simulink model "original_sim_bandpass_singleBand"  (R2024b)
settings: Solver=FixedStepDiscrete  StartTime=0.0  StopTime=(size(sm_EEG_data,1)-1)/sm.p.EEG.sr  RelTol=1e-3  EnableMultiTasking=on
values from neighbouring files (symbols this model uses):
  sm =     [reference_output.mat]
undefined symbols (not defined in the file or in its folder): fdesignblkfcn, gcbh
libraries: dspsrcs4 x1
settings Model: Creator=ronens  LastModifiedBy=hardeep
settings SolverCC: AlgebraicLoopSolver=TrustRegion
settings DataIOCC: LimitDataPoints=on  SaveFormat=Array  SignalLoggingSaveFormat=ModelDataLogs  ReturnWorkspaceOutputs=off
settings OptimizationCC: ExpressionDepthLimit=2147483647  LifeSpan=inf
settings DebuggingCC: UnderspecifiedInitializationDetection=Classic  MergeDetectMultiDrivingBlocksExec=none  SolverPrmCheckMsg=warning  ParameterPrecisionLossMsg=none  FcnCallInpInsideContextMsg=warning  UnconnectedInputMsg=warning  UnconnectedOutputMsg=warning  UnconnectedLineMsg=warning  StateNameClashWarn=warning  SFUnexpectedBacktrackingDiag=warning  SFNoUnconditionalDefaultTransitionDiag=warning  SFExecutionAtInitializationDiag=none  ArithmeticOperatorsInVariantConditions=warning
settings HardwareCC: ProdBitPerPointer=32  ProdBitPerSizeT=32  ProdBitPerPtrDiffT=32  ProdLargestAtomicFloat=None  ProdIntDivRoundTo=Undefined  ProdEndianess=Unspecified  ProdWordSize=32  ProdHWDeviceType=32-bit Generic
settings ModelReferenceCC: EnableRefExpFcnMdlSchedulingChecks=on  PropagateSignalLabelsOutOfModel=off
settings SFSimCC: SimUseLocalCustomCode=off  CustomCodeUndefinedFunction=UseInterfaceOnly
settings RTWCC: RTWUseLocalCustomCode=off  GPUComputeCapability=3.5
settings CodeAppCC: StateflowObjectComments=on
settings GRTTargetCC: TargetLangStandard=C89/C90 (ANSI)
settings ConfigComp: CovMetricSettings=dw  CovSaveCumulativeToWorkspaceVar=on  CovSaveSingleToWorkspaceVar=on  CovExternalEMLEnable=off
settings SimscapeCC: SimscapeNormalizeSystem=off
settings ConfigurationSet: Description=SimMechanics 2G

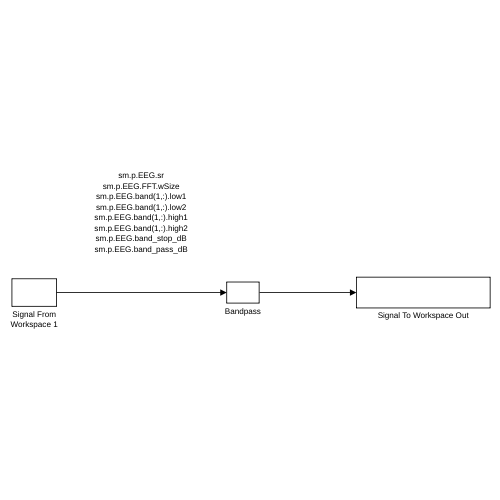
[thumbnail: Simulink's stored preview of the top-level diagram]
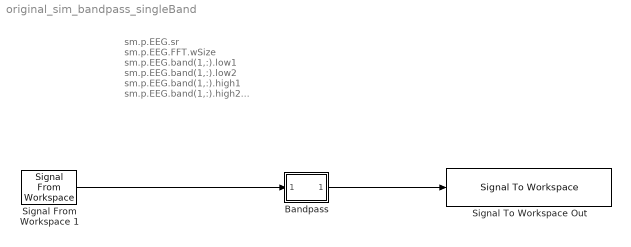
== system original_sim_bandpass_singleBand ==
  note: sm.p.EEG.sr
      | sm.p.EEG.FFT.wSize
      | sm.p.EEG.band(1,:).low1
      | sm.p.EEG.band(1,:).low2
      | sm.p.EEG.band(1,:).high1
      | sm.p.EEG.band(1,:).high2
      | sm.p.EEG.band_stop_dB
      | sm.p.EEG.band_pass_dB
  Bandpass : Subsystem
  Signal From Workspace 1 : dspsrcs4/Signal From Workspace  X=sm_EEG_data  Ts=1/sm.p.EEG.sr  nsamps=1  OutputAfterFinalValue=Setting to zero  ignoreOrWarnInputAndFrameLengths=off  OutputFrames=on
  Signal To Workspace Out : SignalToWorkspace  VariableName=Bandpass_singleBand
      settings: CopyFcn=dspblkcopystw(gcbh);
  wires:
  Signal From Workspace 1/1 -> Bandpass/1(In1)
  Bandpass/1(Out1) -> Signal To Workspace Out/1

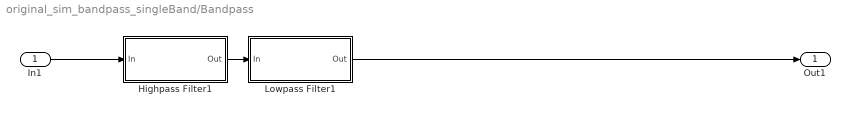
== system original_sim_bandpass_singleBand/Bandpass ==
  In1 : Inport
  Highpass Filter1 : Subsystem  DialogController=fdesignblkfcn  InitFcn=fdesignblkfcn(gcbh, {'InitFcn'});  mask(Highpass Filter){}
      mask help: Design a highpass filter
      settings: CopyFcn=fdesignblkfcn(gcbh, {'CopyFcn'});
      mask Help: helpview(mapfilelocation('dsp'), 'dsphighpassfilter');
      mask Display: disp('Highpass')
  Lowpass Filter1 : Subsystem  DialogController=fdesignblkfcn  InitFcn=fdesignblkfcn(gcbh, {'InitFcn'});  mask(Lowpass Filter){}
      mask help: Design a lowpass filter
      settings: CopyFcn=fdesignblkfcn(gcbh, {'CopyFcn'});
      mask Help: helpview(mapfilelocation('dsp'), 'dsplowpassfilter');
      mask Display: disp('Lowpass')
  Out1 : Outport
  wires:
  In1/1 -> Highpass Filter1/1(In)
  Highpass Filter1/1(Out) -> Lowpass Filter1/1(In)
  Lowpass Filter1/1(Out) -> Out1/1

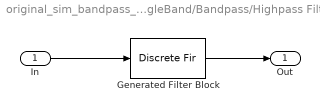
== system original_sim_bandpass_singleBand/Bandpass/Highpass Filter1 ==
  In : Inport
  Generated Filter Block : DiscreteFir  Tag=BlockMethodSubSystem  Coefficients=[-0.00840141778639717091 0.0173152224167967689 0.00308884947939271895 -0.00256762501130670907 -0.00423142192173075072 -0.00412026657980465571 -0.00329310593463389128 -0.002262732561662414 -0.00125968485465549444 -0.000392684840722325548 0.000304955573172563323 0.000822116755893660938 0.00117292528572729925 0.00137046595797921263 0.00144020225152880648 0.00139972588165432278 0.00127632771193091879 0.00108595288663199075 0.000854103588177903888 0.000594267545754096531 0.000327694684087062886 6.38551808909070077e-05 -0.000179450724560961872 -0.000397874081475507052 -0.000577963879948238429 -0.000719776889684668048 -0.000814672778546917699 -0.000866690567111298824 -0.000870392468345223169 -0.000834408096741966242 -0.000756342536848797205 -0.000647695094384184711 -0.000508513373527671726 -0.000352052829416214417 -0.000179389813557604598 -6.03349057744724519e-06 0.000167995555248989494 0.000327549877530480251 0.000473373899657685937 0.000591363324463213482 0.000685218342133664306 0.000741329035878340653 0.000768585479969400827 0.000753109204614785797 0.000709989097617417142 0.000626074902749358566 0.000518403169583120838 0.000387532180141191625 0.000223486800967541188 8.11274228046873498e-05 -0.000115389367192012801 -0.00025834783697307155 -0.000417485752251392625 -0.000565245925697868646 -0.000663489424197992125 -0.000742195313648855441 -0.000802778125940541609 -0.000807484686633235427 -0.000770219657810799476 -0.000711631558497011012 -0.000619998931755313823 -0.000483050872794562052 -0.000321413988640333764 -0.000153717015526360409 2.27220941756313879e-05 0.000210824767849350427 0.00039636524325277955 0.00055828007153160364 0.000690912002654363614 0.000797140998280385224 0.000875342473615355683 0.000912254358274695756 0.000900890166260798642 0.0008416310845922925 0.000745167556431057293 0.000616216536435795249 0.000457526778234206011 0.000268148897373869123 5.91646691704717247e-05 -0.000157866268265354696 -0.000366404857881273585 -0.000559796517825759368 -0.000730065774504567153 -0.00087460992705030321 -0.000981106285025435797 -0.00104421636832933225 -0.00105372525111916641 -0.00101210867575669741 -0.000919233909846757058 -0.000785414510046180542 -0.000610381701853770532 -0.000406780191843504548 -0.000173303851576987235 7.20373868736900541e-05 0.00032448590556910246 0.000564583909527311334 0.000778948373045466164 0.000965020151494673387 0.00109860528816741799 0.00119531980427785246 0.00122974161480201953 0.00120996458749239762 0.00113578507003964688 0.000997595080588046645 0.00080991362702319302 0.000580730320013465276 0.000313104306345794953 2.7668199553746984e-05 -0.000260607543396719867 -0.00054613423249910871 -0.000812759539448379875 -0.00104353866549433054 -0.00123218715350877236 -0.00137044349611684102 -0.00144309434064109434 -0.00144615789305872289 -0.00138121076942770179 -0.0012489288980708326 -0.001050081849674757 -0.000796785231903415791 -0.000502178253391383873 -0.000178960051172325933 0.000163224766678344001 0.000505737826522577186 0.000830861151816729448 0.00112283471959526409 0.00137186034084307829 0.00156132287412795532 0.00167952107584457954 0.00171702472149959785 0.00167415493664422785 0.00154974850149049224 0.001348980083380775 0.00107592528674645875 0.000746673324626800808 0.000374655135267273995 -2.16159478310621574e-05 -0.00042863836990482667 -0.000824381222395672306 -0.00119351166901265969 -0.00151019214123175919 -0.00176512000639446917 -0.00193998548851638465 -0.00202938824178094555 -0.00202275738797201652 -0.001915866871585006 -0.0017167889668052343 -0.00142672770768961441 -0.0010660049780923872 -0.000644129787264740715 -0.000178970697292878822 0.000303711730957656944 0.000786656921706672301 0.00124129009773345689 0.001646399374701221 0.00198576971536819531 0.00223936228102286162 0.00239129921621168522 0.00243491905326593009 0.0023616376574131224 0.0021716729037668729 0.0018740983339220643 0.00148042770867760128 0.00100322029275638921 0.0004662268872081259 -0.000107610602182091865 -0.000692898192660682281 ...(+8639 chars)]  InputProcessing=Columns as channels (frame based)
  Out : Outport
  wires:
  Generated Filter Block/1 -> Out/1
  In/1 -> Generated Filter Block/1

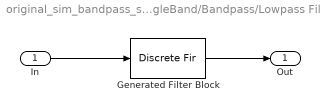
== system original_sim_bandpass_singleBand/Bandpass/Lowpass Filter1 ==
  In : Inport
  Generated Filter Block : DiscreteFir  Tag=BlockMethodSubSystem  Coefficients=[-0.000708660590140460325 -0.000516036018267229083 -0.000676218484847607073 -0.000845253078355269125 -0.00101476002259025147 -0.00117535064458045772 -0.00131640532012708075 -0.00142742693244584176 -0.00149794084506556235 -0.00151885083948529484 -0.00148232013264117547 -0.00138328107406107182 -0.00121936646770160893 -0.000992226480982603487 -0.000706764436244738492 -0.000371677086615355241 1.70027901321316245e-06 0.000398581994929900142 0.000802130972550262294 0.00119370244251402937 0.00155563846000986573 0.00187071110973724528 0.00212341994031031624 0.00230028023929300428 0.00239441659065529715 0.00240139662293428584 0.0023212084097573968 0.00216184746067343012 0.00193220704661738922 0.00164839131449892097 0.00132787252298747203 0.000991401852807027948 0.000659887321213660548 0.000354054725702884147 9.24669306795675839e-05 -0.000109200369526485377 -0.000239669577548094715 -0.000292752995234886113 -0.000267874472634878477 -0.000169885987488796317 -8.7935724770836792e-06 0.000200738308084739335 0.000440519921259248035 0.000690312128903728295 0.000929401182660368006 0.00113760455417379644 0.00129727670408939441 0.0013946317307601435 0.00142063695279547714 0.00137129310245833456 0.00124944686687294103 0.00106278274302946843 0.000824474680769206043 0.000552071252138416056 0.000265482992553120738 -1.34041381388326353e-05 -0.000263633470996998119 -0.0004659116809227784 -0.000604755580447864692 -0.000669254772356847735 -0.000654417868232474 -0.000561408698399622967 -0.000397663766304554294 -0.000176246321867021526 8.49427993368594668e-05 0.000364565854944075892 0.000639565527034913141 0.000886944883985683343 0.00108548160570667265 0.00121758564724780719 0.00127091116655530926 0.00123910503647427792 0.00112256720993266076 0.000928703470113043019 0.000671303483341051908 0.000369348937883060902 4.6210212851065149e-05 -0.000273069400807709529 -0.000562852307528251532 -0.000799565213519618781 -0.000963459671006351021 -0.00104019322599633842 -0.00102228752594939903 -0.000909665399783763425 -0.000710019446549307073 -0.000438147029507722605 -0.00011503338712761723 0.000233763160066979397 0.000580033163851450618 0.000895250924616002031 0.00115283179146867271 0.00133023002060071076 0.00141096266986717755 0.00138611745917859496 0.00125513469904990215 0.00102603768172597411 0.000715115968525232995 0.000345602765219237777 -5.39880850387177317e-05 -0.000451972089260153334 -0.000816145445567714668 -0.00111637950688225017 -0.00132686265454443238 -0.00142879534898759171 -0.00141147273518956741 -0.00127385826062181048 -0.00102453349066569557 -0.00068146554692099712 -0.000270591714210885351 0.000176035902392977729 0.000622715191464168444 0.00103287943190906537 0.00137212943281598719 0.0016110418097759645 0.00172766114928077971 0.00170945789166512753 0.00155466066598262888 0.00127250608614333819 0.000882860301753107162 0.000414834399978641509 -9.5378841359834471e-05 -0.000607332103342868258 -0.00107937709177274074 -0.0014721899547527088 -0.0017519248171356575 -0.0018930813865415026 -0.0018809080490769293 -0.00171277771794879131 -0.00139860548586007074 -0.000960607028096735266 -0.000431454074226722648 0.000147767216683177298 0.000731056351950076832 0.00127080375607802228 0.00172186328427481562 0.00204511912790925282 0.00221097644160241297 0.0022018380587423619 0.00201399888707437654 0.0016582028859886955 0.00115918586326689186 0.000553929150771374106 -0.000110885691116254821 -0.000782606016839246937 -0.00140659291465701736 -0.00193071880861246832 -0.00230961838824543216 -0.00250863603812357836 -0.00250676951146132018 -0.00229894613823932153 -0.00189670700888282077 -0.00132773891257075959 -0.000634102532609447209 0.000130859654158686626 0.000906579572437582275 0.0016298974353042635 0.00224031404795348209 0.00268474084793599065 0.00292231480389681031 0.00292779313650843838 0.00269425697827155178 0.00223398386707575249 0.00157820904543768347 0.000774895804288281104 -0.000114507646182581476 -0.00101982382503595773 -0.00186749482490713146 ...(+7954 chars)]  InputProcessing=Columns as channels (frame based)
  Out : Outport
  wires:
  In/1 -> Generated Filter Block/1
  Generated Filter Block/1 -> Out/1
